simulink model "EZEStateCtrl"  (R2018b)
settings: Solver=FixedStepDiscrete  StartTime=0.0  StopTime=10.0  FixedStep=0.01  RelTol=1e-3
libraries: StateCtrlLib x1
settings Model: Creator=sn2xws  LastModifiedBy=sn2xws
settings DataIOCC: SaveFormat=StructureWithTime
settings OptimizationCC: DefaultParameterBehavior=Inlined  EnhancedBackFolding=on  PassReuseOutputArgsAs=Individual arguments  ZeroExternalMemoryAtStartup=off  ZeroInternalMemoryAtStartup=off  OptimizeBlockOrder=speed  DifferentSizesBufferReuse=on  OptimizationCustomize=off
settings DebuggingCC: ParameterTunabilityLossMsg=error
settings ModelReferenceCC: ModelReferenceNumInstancesAllowed=Single
settings SFSimCC: MATLABDynamicMemAlloc=off
settings RTWCC: SystemTargetFile=autosar.tlc  GenCodeOnly=on  TemplateMakefile=ert_default_tmf  Description=AUTOSAR  GenerateReport=on  IncludeHyperlinkInReport=on  LaunchReport=on  GenerateTraceInfo=on  GenerateTraceReport=on  GenerateTraceReportSl=on  GenerateTraceReportSf=on  GenerateTraceReportEml=on
settings CodeAppCC: ForceParamTrailComments=on  IgnoreCustomStorageClasses=off  OperatorAnnotations=on  SimulinkDataObjDesc=on  SFDataObjDesc=on  InsertBlockDesc=on
settings STFCustomTargetCC: TargetLangStandard=C99 (ISO)  MultiwordLength=256  ParMdlRefBuildCompliant=on  CompOptLevelCompliant=on  IncludeMdlTerminateFcn=off  CombineOutputUpdateFcns=on  SuppressErrorStatus=on  ERTCustomFileBanners=on  SupportNonFinite=off  SupportComplex=off  SupportContinuousTime=off  SupportNonInlinedSFcns=off  RemoveResetFunc=on  MATLABClassNameForMDSCustomization=Simulink.SoftwareTarget.ERTCustomization  AutosarCompliant=on  UseToolchainInfoCompliant=on  LookupTableObjectStructAxisOrder=2,1,3,4,...  LUTObjectStructOrderEvenSpacing=Size,Table,Breakpoints  SystemTargetFile=autosar.tlc
settings ERTTargetCC: TargetLangStandard=C99 (ISO)  ConcurrentExecutionCompliant=off  IncludeMdlTerminateFcn=off  SuppressErrorStatus=on  SupportNonFinite=off  SupportComplex=off  ModelStepFunctionPrototypeControlCompliant=off  CPPClassGenCompliant=off  AutosarCompliant=on  LookupTableObjectStructAxisOrder=2,1,3,4,...  LUTObjectStructOrderEvenSpacing=Size,Table,Breakpoints  InlinedParameterPlacement=NonHierarchical  ERTCustomFileTemplate=example_file_process.tlc

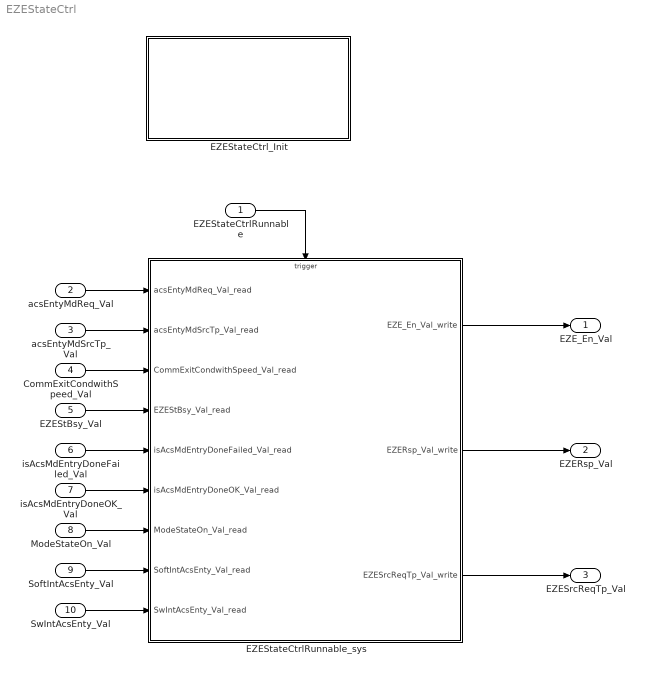
== system EZEStateCtrl ==
  EZEStateCtrlRunnable : Inport  SampleTime=0.01  OutputFunctionCall=on
  acsEntyMdReq_Val : Inport  Port=2  OutDataTypeStr=boolean  PortDimensions=1
  acsEntyMdSrcTp_Val : Inport  Port=3  OutDataTypeStr=Enum: SrcReqTp1  PortDimensions=1
  CommExitCondwithSpeed_Val : Inport  Port=4  OutDataTypeStr=boolean  PortDimensions=1
  EZEStBsy_Val : Inport  Port=5  OutDataTypeStr=boolean  PortDimensions=1
  isAcsMdEntryDoneFailed_Val : Inport  Port=6  OutDataTypeStr=boolean  PortDimensions=1
  isAcsMdEntryDoneOK_Val : Inport  Port=7  OutDataTypeStr=boolean  PortDimensions=1
  ModeStateOn_Val : Inport  Port=8  OutDataTypeStr=boolean  PortDimensions=1
  SoftIntAcsEnty_Val : Inport  Port=9  OutDataTypeStr=IntEnable  PortDimensions=1
  SwIntAcsEnty_Val : Inport  Port=10  OutDataTypeStr=IntEnable  PortDimensions=1
  EZEStateCtrlRunnable_sys : Subsystem
  EZEStateCtrl_Init : Subsystem
  EZE_En_Val : Outport  OutDataTypeStr=boolean  PortDimensions=1
  EZERsp_Val : Outport  Port=2  OutDataTypeStr=Enum: MdRspLocal1  PortDimensions=1
  EZESrcReqTp_Val : Outport  Port=3  OutDataTypeStr=Enum: SrcReqTp1  PortDimensions=1
  wires:
  acsEntyMdReq_Val/1 -> EZEStateCtrlRunnable_sys/1(acsEntyMdReq_Val_read)
  acsEntyMdSrcTp_Val/1 -> EZEStateCtrlRunnable_sys/2(acsEntyMdSrcTp_Val_read)
  CommExitCondwithSpeed_Val/1 -> EZEStateCtrlRunnable_sys/3(CommExitCondwithSpeed_Val_read)
  EZEStBsy_Val/1 -> EZEStateCtrlRunnable_sys/4(EZEStBsy_Val_read)
  isAcsMdEntryDoneFailed_Val/1 -> EZEStateCtrlRunnable_sys/5(isAcsMdEntryDoneFailed_Val_read)
  isAcsMdEntryDoneOK_Val/1 -> EZEStateCtrlRunnable_sys/6(isAcsMdEntryDoneOK_Val_read)
  ModeStateOn_Val/1 -> EZEStateCtrlRunnable_sys/7(ModeStateOn_Val_read)
  SoftIntAcsEnty_Val/1 -> EZEStateCtrlRunnable_sys/8(SoftIntAcsEnty_Val_read)
  SwIntAcsEnty_Val/1 -> EZEStateCtrlRunnable_sys/9(SwIntAcsEnty_Val_read)
  EZEStateCtrlRunnable_sys/1(EZE_En_Val_write) -> EZE_En_Val/1
  EZEStateCtrlRunnable_sys/2(EZERsp_Val_write) -> EZERsp_Val/1
  EZEStateCtrlRunnable_sys/3(EZESrcReqTp_Val_write) -> EZESrcReqTp_Val/1
  EZEStateCtrlRunnable/1 -> EZEStateCtrlRunnable_sys/Trigger

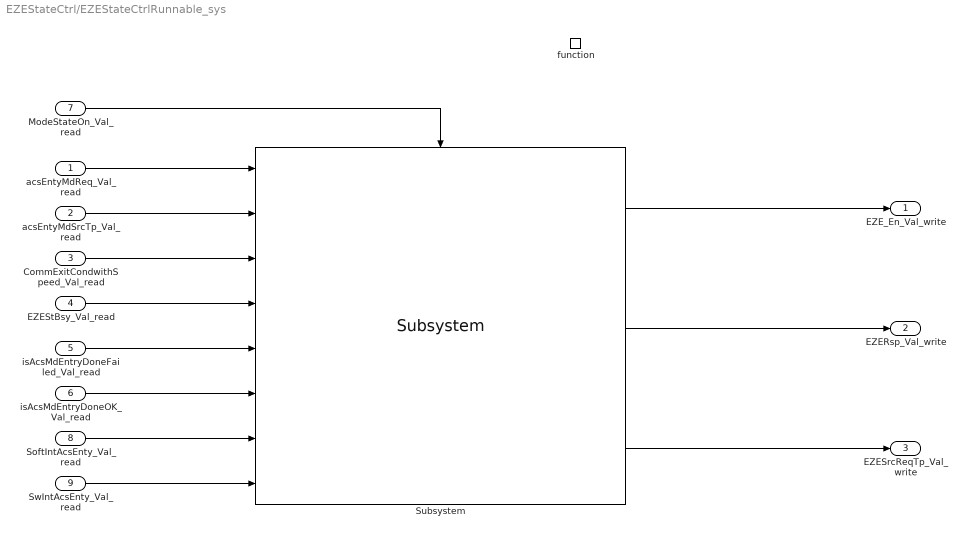
== system EZEStateCtrl/EZEStateCtrlRunnable_sys ==
  acsEntyMdReq_Val_read : Inport
  acsEntyMdSrcTp_Val_read : Inport  Port=2
  CommExitCondwithSpeed_Val_read : Inport  Port=3
  EZEStBsy_Val_read : Inport  Port=4
  isAcsMdEntryDoneFailed_Val_read : Inport  Port=5
  isAcsMdEntryDoneOK_Val_read : Inport  Port=6
  ModeStateOn_Val_read : Inport  Port=7
  SoftIntAcsEnty_Val_read : Inport  Port=8  OutDataTypeStr=IntEnable
  SwIntAcsEnty_Val_read : Inport  Port=9  OutDataTypeStr=IntEnable
  function : TriggerPort  TriggerType=function-call  VariantControl=(inherit)  SampleTimeType=periodic  SampleTime=-1
  Subsystem : StateCtrlLib/Subsystem  SystemSampleTime=-1
  EZE_En_Val_write : Outport
      settings: EnsureOutportIsVirtual=on
  EZERsp_Val_write : Outport  Port=2
      settings: EnsureOutportIsVirtual=on
  EZESrcReqTp_Val_write : Outport  Port=3
      settings: EnsureOutportIsVirtual=on
  wires:
  acsEntyMdReq_Val_read/1 -> Subsystem/1
  acsEntyMdSrcTp_Val_read/1 -> Subsystem/2
  CommExitCondwithSpeed_Val_read/1 -> Subsystem/3
  EZEStBsy_Val_read/1 -> Subsystem/4
  isAcsMdEntryDoneFailed_Val_read/1 -> Subsystem/5
  isAcsMdEntryDoneOK_Val_read/1 -> Subsystem/6
  ModeStateOn_Val_read/1 -> Subsystem/Enable
  SoftIntAcsEnty_Val_read/1 -> Subsystem/7
  SwIntAcsEnty_Val_read/1 -> Subsystem/8
  Subsystem/1 -> EZE_En_Val_write/1
  Subsystem/2 -> EZERsp_Val_write/1
  Subsystem/3 -> EZESrcReqTp_Val_write/1

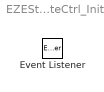
== system EZEStateCtrl/EZEStateCtrl_Init ==
  Event Listener : EventListener  EventName=reset
